simulink model "Condition_Transition_Action"  (R2025b)
settings: Solver=FixedStepDiscrete  StartTime=0.0  StopTime=10.0  FixedStep=0.01  RelTol=1e-3
libraries: simulink x1
settings Model: Creator=soura  LastModifiedBy=soura

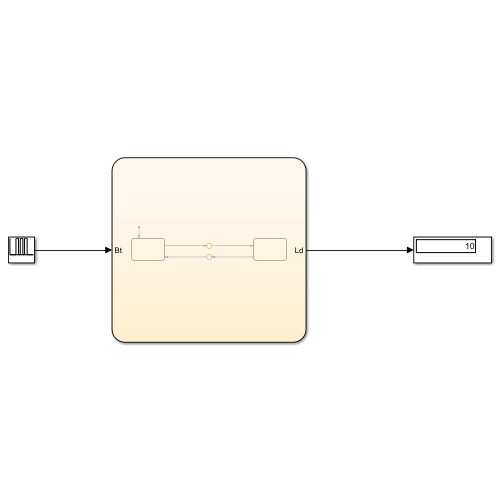
[thumbnail: Simulink's stored preview of the top-level diagram]
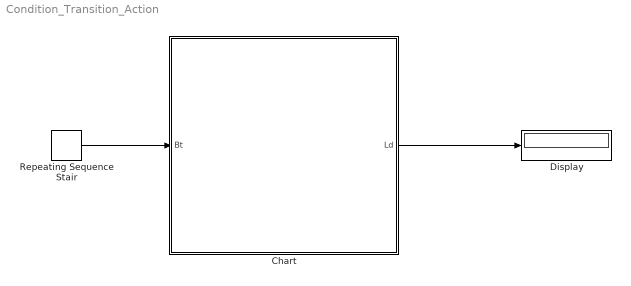
== system Condition_Transition_Action ==
  Chart : Stateflow chart  TreatAsAtomicUnit=on
  Display : Display
  Repeating Sequence Stair : simulink/Sources/Repeating Sequence Stair  OutValues=[0 0 0 0 1 1 0 1 1 0 1 1 0 0 0 0].'  tsamp=-1  OutMin=[]  OutMax=[]  OutDataTypeStr=double  OutputDataTypeScalingMode=double  OutDataType=fixdt(0,8)  ConRadixGroup=Best Precision: Vector-wise  OutScaling=2^-12
  wires:
  Repeating Sequence Stair/1 -> Chart/1(Bt)
  Chart/1(Ld) -> Display/1

== stateflow chart Condition_Transition_Action/Chart ==
  state Off
  state On
    en:
    Ld=1;
  (default) -> Off
  Off -> (junction 14) : %Condition Action
      | [Bt==1]{Ld=0.5;}
  (junction 14) -> On : after(5,tick)
  (junction 8) -> Off : %Transition Action
      | % takes place
      | [Ld==3]
  On -> (junction 8) : %Condition Action
      | [Bt==0]{Ld=Ld+1;}
      | /{Ld=10;}
  data: Bt input; Ld output
